simulink model "multi_opts"  (Simulink 4.00)
settings: Solver=ode45  SolverMode=SingleTasking  StartTime=0  StopTime=5  MaxStep=0.1  RelTol=1e-3  AbsTol=1e-3
libraries: simulink3 x3
(part 1 of 2)
settings Model: LastModifiedBy=mark  Refine=5  SaveTime=off  SaveOutput=off  LimitDataPoints=off  RTWTemplateMakefile=grt_unix.tmf

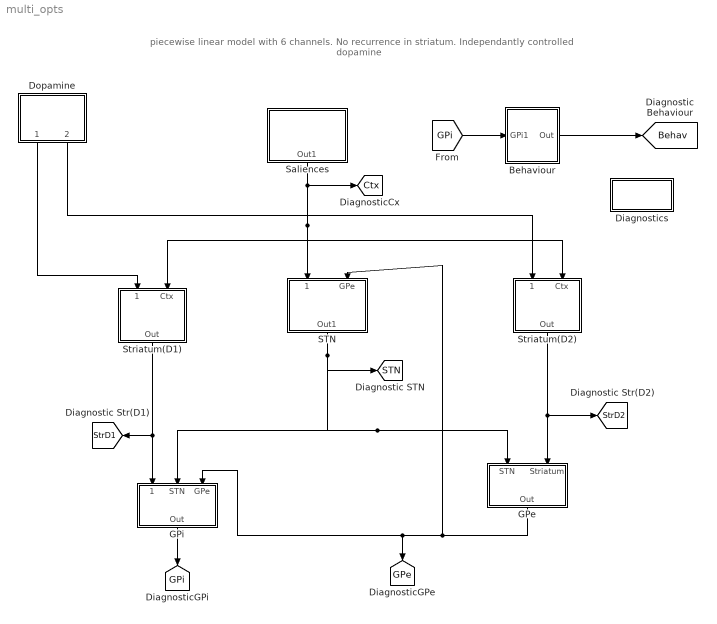
== system multi_opts ==
  note: piecewise linear model with 6 channels. No recurrence in
      | striatum. Independantly controlled dopamine
  Behaviour : Subsystem  mask(Behaviour expression){on_thresh=0.025, off_thresh=0.1}
      mask prompts: on_thresh "GPi level for behav. on"; off_thresh "GPi level for behav.  off"
      settings: RTWFcnNameOpts=Auto  RTWFileNameOpts=Auto
  Diagnostics : Subsystem
      settings: RTWFcnNameOpts=Auto  RTWFileNameOpts=Auto
  Dopamine : Subsystem  Orientation=down
      settings: RTWFcnNameOpts=Auto  RTWFileNameOpts=Auto
  GPe : Subsystem  Orientation=down  mask(GPe){W_str=-1, W_STN=0.8, A_rate=25, slope=1, thresh=-0.2}
      mask prompts: W_str "weight from Striatum"; W_STN "weight from STN (exc.)"; A_rate "membrane decay rate"; slope "output slope"; thresh "output thresh"
      mask help: 3 channel GPe
      settings: RTWFcnNameOpts=Auto  RTWFileNameOpts=Auto
  GPi : Subsystem  Orientation=down  mask(GPi){W_str=-1, W_STN=0.8, W_GPe=-0.4, A_rate=25, slope=1, thresh=-0.2}
      mask prompts: W_str "weight from Str"; W_STN "weight from STN"; W_GPe "weight from GPe"; A_rate "membrane decay rate"; slope "output slope"; thresh "output thresh"
      mask help: 3 channel GPe
      settings: RTWFcnNameOpts=Auto  RTWFileNameOpts=Auto
  STN : Subsystem  Orientation=down
      settings: RTWFcnNameOpts=Auto  RTWFileNameOpts=Auto
  Saliences : Subsystem  Orientation=down
      settings: RTWFcnNameOpts=Auto  RTWFileNameOpts=Auto
  Striatum(D1) : Subsystem  Orientation=down  mask(Striatum (D1)){W_ext=1, A_rate=25, slope=1, thresh=0.2}
      mask prompts: W_ext "External input weight"; A_rate "membrane decay rate"; slope "output slope"; thresh "output thresh"
      mask help: 3 channel striatum - non-recurrent
      settings: RTWFcnNameOpts=Auto  RTWFileNameOpts=Auto
  Striatum(D2) : Subsystem  Orientation=down  mask(Striatum (D1)){W_ext=1, A_rate=25, slope=1, thresh=0.2}
      mask prompts: W_ext "External input weight"; A_rate "membrane decay rate"; slope "output slope"; thresh "output thresh"
      mask help: 3 channel striatum - non-recurrent
      settings: RTWFcnNameOpts=Auto  RTWFileNameOpts=Auto
  tag scope: Behav=global, Ctx=global, GPe=global, GPi=global, STN=global, StrD1=global, StrD2=global
  wires:
  Saliences/1(Out1) -> [Ctx], Striatum(D2)/2(Ctx), Striatum(D1)/2(Ctx), STN/1(salineces)
  [GPi] -> Behaviour/1(GPi1)
  Behaviour/1(Out) -> [Behav]
  GPe/1(Out) -> STN/2(GPe), GPi/3(GPe), [GPe]
  Striatum(D2)/1(Out) -> GPe/2(Striatum), [StrD2]
  STN/1(Out1) -> [STN], GPe/1(STN), GPi/2(STN)
  GPi/1(Out) -> [GPi]
  Striatum(D1)/1(Out) -> GPi/1(Striatum), [StrD1]
  Dopamine/2(GPe(D2)) -> Striatum(D2)/1(Dopamine)
  Dopamine/1(GPi(D1)) -> Striatum(D1)/1(Dopamine)

== system multi_opts/Behaviour ==
  GPi1 : Inport  Port=1  LatchInput=off
  Constant : Constant  Value=1
  Relay : Relay  OnSwitchValue=1 - on_thresh  OffSwitchValue=1 - off_thresh  OnOutputValue=1  OffOutputValue=0
  Sum : Sum  Inputs=+-  SaturateOnIntegerOverflow=on
  Out : Outport  Port=1  InitialOutput=0
  wires:
  Constant/1 -> Sum/1
  Sum/1 -> Relay/1
  GPi1/1 -> Sum/2
  Relay/1 -> Out/1

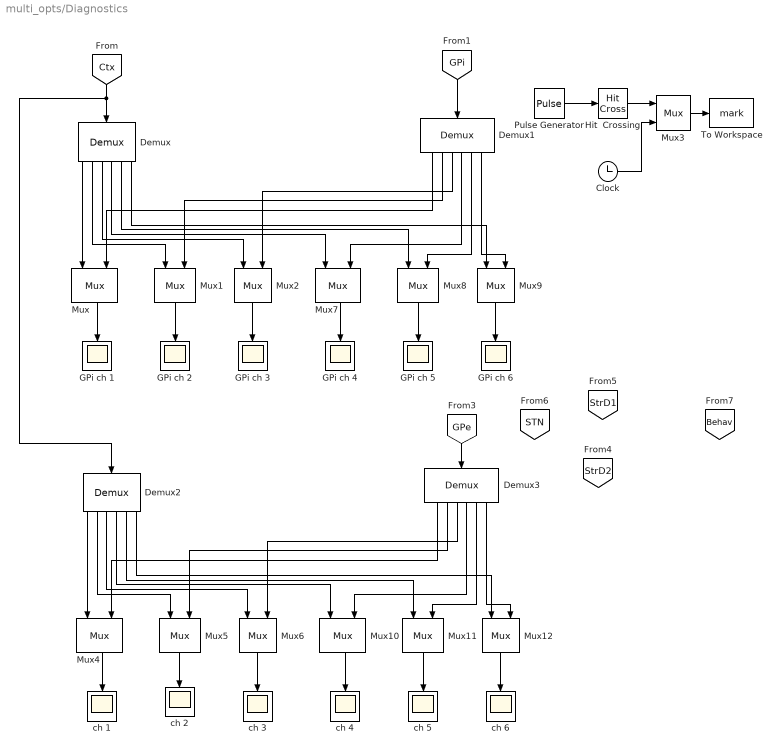
== system multi_opts/Diagnostics ==
  Clock : Clock
      settings: DisplayTime=off  Decimation=10
  Demux{,1..3} (4 alike) : Demux  Orientation=down  Outputs=6  BusSelectionMode=off
  GPi ch {1..6} (6 alike) : Scope
      GPi ch 1 settings: Orientation=down  TickLabels=on  TimeRange=auto  YMin=0  YMax=1  SaveName=GPic1_6  DataFormat=Array  LimitDataPoints=on  MaxDataPoints=7000
      GPi ch 2 settings: Orientation=down  TickLabels=on  TimeRange=auto  YMin=0  YMax=1  SaveName=GPic2_6  DataFormat=Array  LimitDataPoints=on  MaxDataPoints=7000
      GPi ch 3 settings: Orientation=down  TickLabels=on  TimeRange=auto  YMin=0  YMax=1  SaveName=GPic3_6  DataFormat=Array  LimitDataPoints=on  MaxDataPoints=5000
      GPi ch 4 settings: Orientation=down  TickLabels=on  TimeRange=auto  YMin=0  YMax=0.75  SaveToWorkspace=off  SaveName=GPic4_6  DataFormat=Array  LimitDataPoints=on  MaxDataPoints=5000
      GPi ch 5 settings: Orientation=down  TickLabels=on  TimeRange=auto  YMin=0  YMax=0.75  SaveToWorkspace=off  SaveName=GPi3full  DataFormat=Array  LimitDataPoints=on  MaxDataPoints=5000
      GPi ch 6 settings: Orientation=down  TickLabels=on  TimeRange=auto  YMin=0  YMax=0.75  SaveToWorkspace=off  SaveName=GPi6full6  DataFormat=Array  LimitDataPoints=on  MaxDataPoints=5000
  Hit  Crossing : HitCross  HitCrossingOffset=0.5  HitCrossingDirection=falling  ShowOutputPort=on
  Mux{,1..2,4..12} (12 alike) : Mux  Orientation=down  Inputs=2
      settings: DisplayOption=none
  Mux3 : Mux  Inputs=2
      settings: DisplayOption=none
  Pulse Generator : DiscretePulseGenerator  PulseType=Time-based  Amplitude=1  Period=0.5  PulseWidth=50  PhaseDelay=0.0  SampleTime=1
  To Workspace : ToWorkspace  VariableName=mark  SampleTime=-1  SaveFormat=Array
  ch {1..6} (6 alike) : Scope
      ch 1 settings: Orientation=down  TickLabels=on  TimeRange=auto  YMin=0  YMax=1  SaveName=gpe1  DataFormat=Array  LimitDataPoints=on  MaxDataPoints=5000
      ch 2 settings: Orientation=down  TickLabels=on  TimeRange=auto  YMin=0  YMax=0.75  SaveName=gpe2  DataFormat=Array  LimitDataPoints=on  MaxDataPoints=5000
      ch 3 settings: Orientation=down  TickLabels=on  TimeRange=auto  YMin=0  YMax=0.75  SaveToWorkspace=off  SaveName=ch3  DataFormat=Array  LimitDataPoints=on  MaxDataPoints=5000
      ch 4 settings: Orientation=down  TickLabels=on  TimeRange=auto  YMin=0  YMax=0.75  SaveToWorkspace=off  SaveName=ch4  DataFormat=Array  LimitDataPoints=on  MaxDataPoints=5000
      ch 5 settings: Orientation=down  TickLabels=on  TimeRange=auto  YMin=0  YMax=0.75  SaveToWorkspace=off  SaveName=ch5  DataFormat=Array  LimitDataPoints=on  MaxDataPoints=5000
      ch 6 settings: Orientation=down  TickLabels=on  TimeRange=auto  YMin=0  YMax=0.75  SaveToWorkspace=off  SaveName=ch6  DataFormat=Array  LimitDataPoints=on  MaxDataPoints=5000
  wires:
  [GPe] -> Demux3/1
  Mux/1 -> GPi ch 1/1
  Demux/1 -> Mux/1
  Demux/2 -> Mux1/1
  Mux1/1 -> GPi ch 2/1
  Mux2/1 -> GPi ch 3/1
  Demux/3 -> Mux2/1
  Demux/4 -> Mux7/1
  Demux/5 -> Mux8/1
  Demux/6 -> Mux9/1
  Demux1/3 -> Mux2/2
  [GPi] -> Demux1/1
  Demux1/1 -> Mux/2
  Demux1/2 -> Mux1/2
  Demux1/4 -> Mux7/2
  Demux1/5 -> Mux8/2
  Demux1/6 -> Mux9/2
  Mux7/1 -> GPi ch 4/1
  Mux8/1 -> GPi ch 5/1
  Mux9/1 -> GPi ch 6/1
  [Ctx] -> Demux/1, Demux2/1
  Mux4/1 -> ch 1/1
  Demux2/1 -> Mux4/1
  Demux2/2 -> Mux5/1
  Mux5/1 -> ch 2/1
  Mux6/1 -> ch 3/1
  Demux2/3 -> Mux6/1
  Demux2/4 -> Mux10/1
  Demux2/5 -> Mux11/1
  Demux2/6 -> Mux12/1
  Demux3/3 -> Mux6/2
  Demux3/1 -> Mux4/2
  Demux3/2 -> Mux5/2
  Demux3/4 -> Mux10/2
  Demux3/5 -> Mux11/2
  Demux3/6 -> Mux12/2
  Mux10/1 -> ch 4/1
  Mux11/1 -> ch 5/1
  Mux12/1 -> ch 6/1
  Pulse Generator/1 -> Hit  Crossing/1
  Hit  Crossing/1 -> Mux3/1
  Clock/1 -> Mux3/2
  Mux3/1 -> To Workspace/1

== system multi_opts/Dopamine ==
  D1 base level : Constant  Value=0.2
  D2 base level : Constant  Orientation=left  Value=0.2
  Mux : Mux  Orientation=down  Inputs=6
      settings: DisplayOption=none
  Mux1 : Mux  Orientation=down  Inputs=6
      settings: DisplayOption=none
  GPi(D1) : Outport  Orientation=down  Port=1  InitialOutput=0
  GPe(D2) : Outport  Orientation=down  Port=2  InitialOutput=0
  wires:
  Mux1/1 -> GPe(D2)/1
  D2 base level/1 -> Mux1/6, Mux1/5, Mux1/4, Mux1/3, Mux1/2, Mux1/1
  Mux/1 -> GPi(D1)/1
  D1 base level/1 -> Mux/6, Mux/5, Mux/4, Mux/3, Mux/2, Mux/1

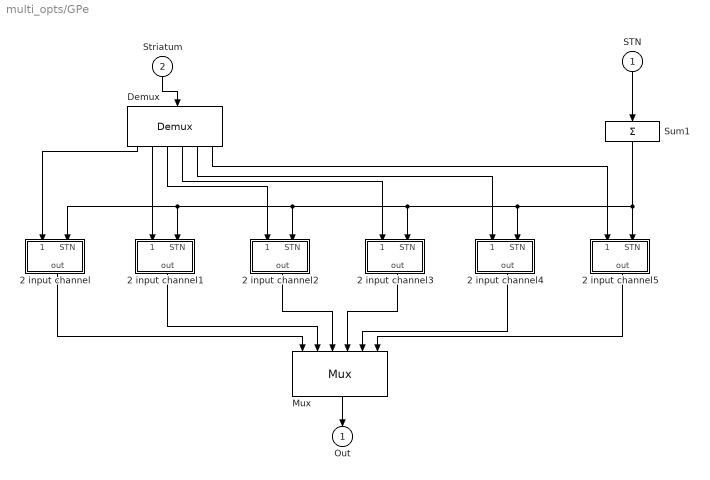
== system multi_opts/GPe ==
  STN : Inport  Orientation=down  Port=1  LatchInput=off
  Striatum : Inport  Orientation=down  Port=2  LatchInput=off
  2 input channel : Subsystem  Orientation=down
      settings: RTWFcnNameOpts=Auto  RTWFileNameOpts=Auto
  2 input channel1 : Subsystem  Orientation=down
      settings: RTWFcnNameOpts=Auto  RTWFileNameOpts=Auto
  2 input channel2 : Subsystem  Orientation=down
      settings: RTWFcnNameOpts=Auto  RTWFileNameOpts=Auto
  2 input channel3 : Subsystem  Orientation=down
      settings: RTWFcnNameOpts=Auto  RTWFileNameOpts=Auto
  2 input channel4 : Subsystem  Orientation=down
      settings: RTWFcnNameOpts=Auto  RTWFileNameOpts=Auto
  2 input channel5 : Subsystem  Orientation=down
      settings: RTWFcnNameOpts=Auto  RTWFileNameOpts=Auto
  Demux : Demux  Orientation=down  Outputs=6  BusSelectionMode=off
  Mux : Mux  Orientation=down  Inputs=6
      settings: DisplayOption=none
  Sum1 : Sum  Orientation=down  Inputs=+  SaturateOnIntegerOverflow=on
  Out : Outport  Orientation=down  Port=1  InitialOutput=0
  wires:
  Sum1/1 -> 2 input channel5/2(STN), 2 input channel/2(STN), 2 input channel1/2(STN), 2 input channel2/2(STN), 2 input channel3/2(STN), 2 input channel4/2(STN)
  Demux/1 -> 2 input channel/1(Striatum)
  STN/1 -> Sum1/1
  2 input channel/1(out) -> Mux/1
  2 input channel1/1(out) -> Mux/2
  2 input channel2/1(out) -> Mux/3
  Mux/1 -> Out/1
  Striatum/1 -> Demux/1
  Demux/2 -> 2 input channel1/1(Striatum)
  Demux/3 -> 2 input channel2/1(Striatum)
  Demux/4 -> 2 input channel3/1(Striatum)
  Demux/5 -> 2 input channel4/1(Striatum)
  Demux/6 -> 2 input channel5/1(Striatum)
  2 input channel3/1(out) -> Mux/4
  2 input channel4/1(out) -> Mux/5
  2 input channel5/1(out) -> Mux/6

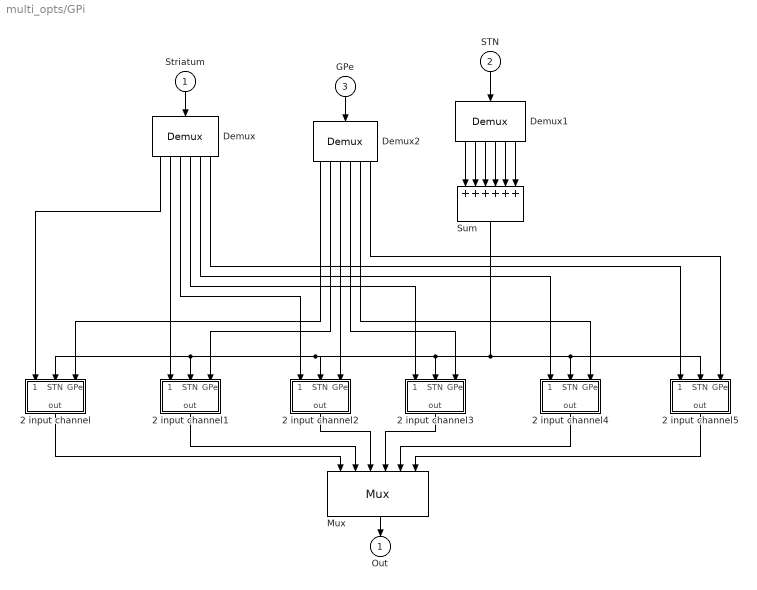
== system multi_opts/GPi ==
  Striatum : Inport  Orientation=down  Port=1  LatchInput=off
  STN : Inport  Orientation=down  Port=2  LatchInput=off
  GPe : Inport  Orientation=down  Port=3  LatchInput=off
  2 input channel : Subsystem  Orientation=down
      settings: RTWFcnNameOpts=Auto  RTWFileNameOpts=Auto
  2 input channel1 : Subsystem  Orientation=down
      settings: RTWFcnNameOpts=Auto  RTWFileNameOpts=Auto
  2 input channel2 : Subsystem  Orientation=down
      settings: RTWFcnNameOpts=Auto  RTWFileNameOpts=Auto
  2 input channel3 : Subsystem  Orientation=down
      settings: RTWFcnNameOpts=Auto  RTWFileNameOpts=Auto
  2 input channel4 : Subsystem  Orientation=down
      settings: RTWFcnNameOpts=Auto  RTWFileNameOpts=Auto
  2 input channel5 : Subsystem  Orientation=down
      settings: RTWFcnNameOpts=Auto  RTWFileNameOpts=Auto
  Demux : Demux  Orientation=down  Outputs=6  BusSelectionMode=off
  Demux1 : Demux  Orientation=down  Outputs=6  BusSelectionMode=off
  Demux2 : Demux  Orientation=down  Outputs=6  BusSelectionMode=off
  Mux : Mux  Orientation=down  Inputs=6
      settings: DisplayOption=none
  Sum : Sum  Orientation=down  Inputs=++++++  SaturateOnIntegerOverflow=on
  Out : Outport  Orientation=down  Port=1  InitialOutput=0
  wires:
  Mux/1 -> Out/1
  2 input channel2/1(out) -> Mux/3
  2 input channel1/1(out) -> Mux/2
  2 input channel/1(out) -> Mux/1
  GPe/1 -> Demux2/1
  Demux2/1 -> 2 input channel/3(GPe)
  Demux2/2 -> 2 input channel1/3(GPe)
  Demux2/3 -> 2 input channel2/3(GPe)
  Demux/2 -> 2 input channel1/1(Striatum)
  Demux/1 -> 2 input channel/1(Striatum)
  Striatum/1 -> Demux/1
  Demux/3 -> 2 input channel2/1(Striatum)
  Demux/4 -> 2 input channel3/1(Striatum)
  Demux/5 -> 2 input channel4/1(Striatum)
  Demux/6 -> 2 input channel5/1(Striatum)
  Demux2/4 -> 2 input channel3/3(GPe)
  Demux2/5 -> 2 input channel4/3(GPe)
  Demux1/1 -> Sum/1
  Demux1/2 -> Sum/2
  Demux1/3 -> Sum/3
  Demux1/4 -> Sum/4
  Demux1/5 -> Sum/5
  Demux1/6 -> Sum/6
  STN/1 -> Demux1/1
  Sum/1 -> 2 input channel/2(STN), 2 input channel1/2(STN), 2 input channel2/2(STN), 2 input channel3/2(STN), 2 input channel4/2(STN), 2 input channel5/2(STN)
  Demux2/6 -> 2 input channel5/3(GPe)
  2 input channel3/1(out) -> Mux/4
  2 input channel4/1(out) -> Mux/5
  2 input channel5/1(out) -> Mux/6

== system multi_opts/STN ==
  salineces : Inport  Orientation=down  Port=1  LatchInput=off
  GPe : Inport  Orientation=down  Port=2  LatchInput=off
  Do discrete STN : Constant  Orientation=down  Value=1
  STN discrete model : Subsystem  Orientation=down  mask(STN){W_ctx=1, W_GPe=-1, A_rate=25, slope=1, thresh=-0.25}
      mask prompts: W_ctx "weight from Cortex"; W_GPe "weight from GPe(inhib.)"; A_rate "membrane decay rate"; slope "output slope"; thresh "output thresh"
      mask help: 3 channel GPe
      settings: RTWFcnNameOpts=Auto  RTWFileNameOpts=Auto
  STN homogeneous model : Subsystem  Orientation=down  mask(STN){epsilon_p=0.25, W_ctx=1, W_GPe=-1, A_rate=25, slope=1, thresh=0}
      mask prompts: epsilon_p "Ctx tonic rate (per channel)"; W_ctx "weight from Ctx"; W_GPe "weight from GPe(inhib.)"; A_rate "membrane decay rate"; slope "output slope"; thresh "output thresh"
      mask help: 3 channel GPe
      settings: RTWFcnNameOpts=Auto  RTWFileNameOpts=Auto
  Switch1 : Switch  Orientation=down  Threshold=0.5
  Out1 : Outport  Orientation=down  Port=1  InitialOutput=0
  wires:
  STN homogeneous model/1(Out) -> Switch1/3
  GPe/1 -> STN discrete model/2(GPe), STN homogeneous model/2(GPe)
  salineces/1 -> STN homogeneous model/1(Cortex), STN discrete model/1(Cortex)
  Switch1/1 -> Out1/1
  Do discrete STN/1 -> Switch1/2
  STN discrete model/1(Out) -> Switch1/1

== system multi_opts/Saliences ==
  Do left : Constant  Orientation=down  Value=0
  Salience (simple) : Subsystem  Orientation=down
      settings: RTWFcnNameOpts=Auto  RTWFileNameOpts=Auto
  Switch : Switch  Orientation=down  Threshold=0.5
  step pairs : Subsystem  Orientation=down
      settings: RTWFcnNameOpts=Auto  RTWFileNameOpts=Auto
  Out1 : Outport  Orientation=down  Port=1  InitialOutput=0
  wires:
  Switch/1 -> Out1/1
  Salience (simple)/1(out) -> Switch/3
  step pairs/1(out) -> Switch/1
  Do left/1 -> Switch/2

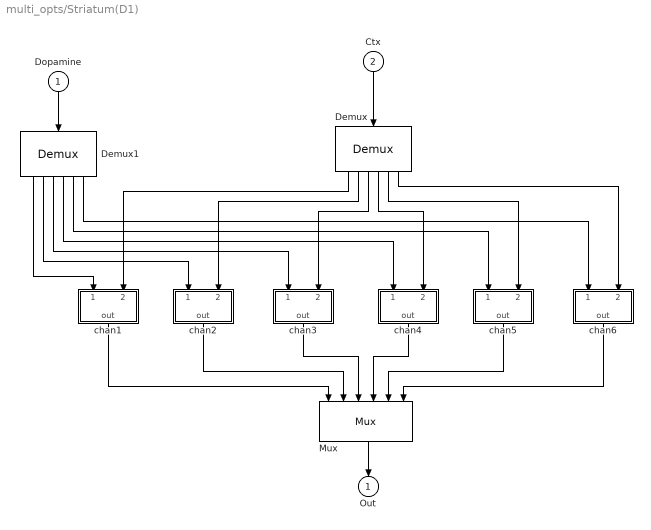
== system multi_opts/Striatum(D1) ==
  Dopamine : Inport  Orientation=down  Port=1  LatchInput=off
  Ctx : Inport  Orientation=down  Port=2  LatchInput=off
  Demux : Demux  Orientation=down  Outputs=6  BusSelectionMode=off
  Demux1 : Demux  Orientation=down  Outputs=6  BusSelectionMode=off
  Mux : Mux  Orientation=down  Inputs=6
      settings: DisplayOption=none
  chan1 : Subsystem  Orientation=down
      settings: RTWFcnNameOpts=Auto  RTWFileNameOpts=Auto
  chan2 : Subsystem  Orientation=down
      settings: RTWFcnNameOpts=Auto  RTWFileNameOpts=Auto
  chan3 : Subsystem  Orientation=down
      settings: RTWFcnNameOpts=Auto  RTWFileNameOpts=Auto
  chan4 : Subsystem  Orientation=down
      settings: RTWFcnNameOpts=Auto  RTWFileNameOpts=Auto
  chan5 : Subsystem  Orientation=down
      settings: RTWFcnNameOpts=Auto  RTWFileNameOpts=Auto
  chan6 : Subsystem  Orientation=down
      settings: RTWFcnNameOpts=Auto  RTWFileNameOpts=Auto
  Out : Outport  Orientation=down  Port=1  InitialOutput=0
  wires:
  Ctx/1 -> Demux/1
  Mux/1 -> Out/1
  chan1/1(out) -> Mux/1
  chan3/1(out) -> Mux/3
  chan2/1(out) -> Mux/2
  Demux/1 -> chan1/2(external)
  Demux/2 -> chan2/2(external)
  Demux/3 -> chan3/2(external)
  Demux/4 -> chan4/2(external)
  Demux/5 -> chan5/2(external)
  Demux/6 -> chan6/2(external)
  chan4/1(out) -> Mux/4
  chan5/1(out) -> Mux/5
  chan6/1(out) -> Mux/6
  Dopamine/1 -> Demux1/1
  Demux1/6 -> chan6/1(dopamine)
  Demux1/5 -> chan5/1(dopamine)
  Demux1/4 -> chan4/1(dopamine)
  Demux1/3 -> chan3/1(dopamine)
  Demux1/2 -> chan2/1(dopamine)
  Demux1/1 -> chan1/1(dopamine)

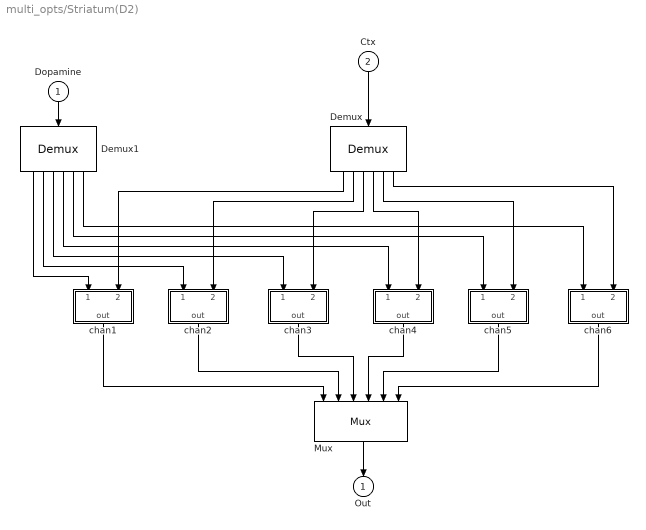
== system multi_opts/Striatum(D2) ==
  Dopamine : Inport  Orientation=down  Port=1  LatchInput=off
  Ctx : Inport  Orientation=down  Port=2  LatchInput=off
  Demux : Demux  Orientation=down  Outputs=6  BusSelectionMode=off
  Demux1 : Demux  Orientation=down  Outputs=6  BusSelectionMode=off
  Mux : Mux  Orientation=down  Inputs=6
      settings: DisplayOption=none
  chan1 : Subsystem  Orientation=down
      settings: RTWFcnNameOpts=Auto  RTWFileNameOpts=Auto
  chan2 : Subsystem  Orientation=down
      settings: RTWFcnNameOpts=Auto  RTWFileNameOpts=Auto
  chan3 : Subsystem  Orientation=down
      settings: RTWFcnNameOpts=Auto  RTWFileNameOpts=Auto
  chan4 : Subsystem  Orientation=down
      settings: RTWFcnNameOpts=Auto  RTWFileNameOpts=Auto
  chan5 : Subsystem  Orientation=down
      settings: RTWFcnNameOpts=Auto  RTWFileNameOpts=Auto
  chan6 : Subsystem  Orientation=down
      settings: RTWFcnNameOpts=Auto  RTWFileNameOpts=Auto
  Out : Outport  Orientation=down  Port=1  InitialOutput=0
  wires:
  chan6/1(out) -> Mux/6
  chan5/1(out) -> Mux/5
  chan4/1(out) -> Mux/4
  Demux/6 -> chan6/2(external)
  Demux/5 -> chan5/2(external)
  Demux/4 -> chan4/2(external)
  Demux/3 -> chan3/2(external)
  Demux/2 -> chan2/2(external)
  Demux/1 -> chan1/2(external)
  chan2/1(out) -> Mux/2
  chan3/1(out) -> Mux/3
  chan1/1(out) -> Mux/1
  Mux/1 -> Out/1
  Ctx/1 -> Demux/1
  Dopamine/1 -> Demux1/1
  Demux1/6 -> chan6/1(dopamine)
  Demux1/5 -> chan5/1(dopamine)
  Demux1/4 -> chan4/1(dopamine)
  Demux1/3 -> chan3/1(dopamine)
  Demux1/2 -> chan2/1(dopamine)
  Demux1/1 -> chan1/1(dopamine)

== system multi_opts/GPe/2 input channel ==
  Striatum : Inport  Orientation=down  Port=1  LatchInput=off
  STN : Inport  Orientation=down  Port=2  LatchInput=off
  input summation : Subsystem  Orientation=down
      settings: RTWFcnNameOpts=Auto  RTWFileNameOpts=Auto
  leaky integration : Subsystem  Orientation=down
      settings: RTWFcnNameOpts=Auto  RTWFileNameOpts=Auto
  piecewise lin. : S-Function  Orientation=down  FunctionName=Mpieclin  Parameters=slope,thresh  PortCounts=[]  SFunctionModules=''
  out : Outport  Orientation=down  Port=1  InitialOutput=0
  wires:
  leaky integration/1(Outport) -> piecewise lin./1
  input summation/1(out_1) -> leaky integration/1(Inport)
  Striatum/1 -> input summation/1(x1)
  STN/1 -> input summation/2(x2)
  piecewise lin./1 -> out/1

== system multi_opts/GPe/2 input channel1 ==
  Striatum : Inport  Orientation=down  Port=1  LatchInput=off
  STN : Inport  Orientation=down  Port=2  LatchInput=off
  input summation : Subsystem  Orientation=down
      settings: RTWFcnNameOpts=Auto  RTWFileNameOpts=Auto
  leaky integration : Subsystem  Orientation=down
      settings: RTWFcnNameOpts=Auto  RTWFileNameOpts=Auto
  piecewise lin. : S-Function  Orientation=down  FunctionName=Mpieclin  Parameters=slope,thresh  PortCounts=[]  SFunctionModules=''
  out : Outport  Orientation=down  Port=1  InitialOutput=0
  wires:
  piecewise lin./1 -> out/1
  STN/1 -> input summation/2(x2)
  Striatum/1 -> input summation/1(x1)
  leaky integration/1(Outport) -> piecewise lin./1
  input summation/1(out_1) -> leaky integration/1(Inport)

== system multi_opts/GPe/2 input channel2 ==
  Striatum : Inport  Orientation=down  Port=1  LatchInput=off
  STN : Inport  Orientation=down  Port=2  LatchInput=off
  input summation : Subsystem  Orientation=down
      settings: RTWFcnNameOpts=Auto  RTWFileNameOpts=Auto
  leaky integration : Subsystem  Orientation=down
      settings: RTWFcnNameOpts=Auto  RTWFileNameOpts=Auto
  piecewise lin. : S-Function  Orientation=down  FunctionName=Mpieclin  Parameters=slope,thresh  PortCounts=[]  SFunctionModules=''
  out : Outport  Orientation=down  Port=1  InitialOutput=0
  wires:
  input summation/1(out_1) -> leaky integration/1(Inport)
  leaky integration/1(Outport) -> piecewise lin./1
  Striatum/1 -> input summation/1(x1)
  STN/1 -> input summation/2(x2)
  piecewise lin./1 -> out/1

== system multi_opts/GPe/2 input channel3 ==
  Striatum : Inport  Orientation=down  Port=1  LatchInput=off
  STN : Inport  Orientation=down  Port=2  LatchInput=off
  input summation : Subsystem  Orientation=down
      settings: RTWFcnNameOpts=Auto  RTWFileNameOpts=Auto
  leaky integration : Subsystem  Orientation=down
      settings: RTWFcnNameOpts=Auto  RTWFileNameOpts=Auto
  piecewise lin. : S-Function  Orientation=down  FunctionName=Mpieclin  Parameters=slope,thresh  PortCounts=[]  SFunctionModules=''
  out : Outport  Orientation=down  Port=1  InitialOutput=0
  wires:
  piecewise lin./1 -> out/1
  STN/1 -> input summation/2(x2)
  Striatum/1 -> input summation/1(x1)
  leaky integration/1(Outport) -> piecewise lin./1
  input summation/1(out_1) -> leaky integration/1(Inport)

== system multi_opts/GPe/2 input channel4 ==
  Striatum : Inport  Orientation=down  Port=1  LatchInput=off
  STN : Inport  Orientation=down  Port=2  LatchInput=off
  input summation : Subsystem  Orientation=down
      settings: RTWFcnNameOpts=Auto  RTWFileNameOpts=Auto
  leaky integration : Subsystem  Orientation=down
      settings: RTWFcnNameOpts=Auto  RTWFileNameOpts=Auto
  piecewise lin. : S-Function  Orientation=down  FunctionName=Mpieclin  Parameters=slope,thresh  PortCounts=[]  SFunctionModules=''
  out : Outport  Orientation=down  Port=1  InitialOutput=0
  wires:
  input summation/1(out_1) -> leaky integration/1(Inport)
  leaky integration/1(Outport) -> piecewise lin./1
  Striatum/1 -> input summation/1(x1)
  STN/1 -> input summation/2(x2)
  piecewise lin./1 -> out/1

== system multi_opts/GPe/2 input channel5 ==
  Striatum : Inport  Orientation=down  Port=1  LatchInput=off
  STN : Inport  Orientation=down  Port=2  LatchInput=off
  input summation : Subsystem  Orientation=down
      settings: RTWFcnNameOpts=Auto  RTWFileNameOpts=Auto
  leaky integration : Subsystem  Orientation=down
      settings: RTWFcnNameOpts=Auto  RTWFileNameOpts=Auto
  piecewise lin. : S-Function  Orientation=down  FunctionName=Mpieclin  Parameters=slope,thresh  PortCounts=[]  SFunctionModules=''
  out : Outport  Orientation=down  Port=1  InitialOutput=0
  wires:
  piecewise lin./1 -> out/1
  STN/1 -> input summation/2(x2)
  Striatum/1 -> input summation/1(x1)
  leaky integration/1(Outport) -> piecewise lin./1
  input summation/1(out_1) -> leaky integration/1(Inport)

== system multi_opts/GPi/2 input channel ==
  Striatum : Inport  Orientation=down  Port=1  LatchInput=off
  STN : Inport  Orientation=down  Port=2  LatchInput=off
  GPe : Inport  Orientation=down  Port=3  LatchInput=off
  input summation : Subsystem  Orientation=down
      settings: RTWFcnNameOpts=Auto  RTWFileNameOpts=Auto
  leaky integration : Subsystem  Orientation=down
      settings: RTWFcnNameOpts=Auto  RTWFileNameOpts=Auto
  piecewise lin. : S-Function  Orientation=down  FunctionName=Mpieclin  Parameters=slope,thresh  PortCounts=[]  SFunctionModules=''
  out : Outport  Orientation=down  Port=1  InitialOutput=0
  wires:
  piecewise lin./1 -> out/1
  STN/1 -> input summation/2(x2)
  Striatum/1 -> input summation/1(x1)
  leaky integration/1(Outport) -> piecewise lin./1
  input summation/1(out_1) -> leaky integration/1(Inport)
  GPe/1 -> input summation/3(x3)

== system multi_opts/GPi/2 input channel1 ==
  Striatum : Inport  Orientation=down  Port=1  LatchInput=off
  STN : Inport  Orientation=down  Port=2  LatchInput=off
  GPe : Inport  Orientation=down  Port=3  LatchInput=off
  input summation : Subsystem  Orientation=down
      settings: RTWFcnNameOpts=Auto  RTWFileNameOpts=Auto
  leaky integration : Subsystem  Orientation=down
      settings: RTWFcnNameOpts=Auto  RTWFileNameOpts=Auto
  piecewise lin. : S-Function  Orientation=down  FunctionName=Mpieclin  Parameters=slope,thresh  PortCounts=[]  SFunctionModules=''
  out : Outport  Orientation=down  Port=1  InitialOutput=0
  wires:
  GPe/1 -> input summation/3(x3)
  input summation/1(out_1) -> leaky integration/1(Inport)
  leaky integration/1(Outport) -> piecewise lin./1
  Striatum/1 -> input summation/1(x1)
  STN/1 -> input summation/2(x2)
  piecewise lin./1 -> out/1

== system multi_opts/GPi/2 input channel2 ==
  Striatum : Inport  Orientation=down  Port=1  LatchInput=off
  STN : Inport  Orientation=down  Port=2  LatchInput=off
  GPe : Inport  Orientation=down  Port=3  LatchInput=off
  input summation : Subsystem  Orientation=down
      settings: RTWFcnNameOpts=Auto  RTWFileNameOpts=Auto
  leaky integration : Subsystem  Orientation=down
      settings: RTWFcnNameOpts=Auto  RTWFileNameOpts=Auto
  piecewise lin. : S-Function  Orientation=down  FunctionName=Mpieclin  Parameters=slope,thresh  PortCounts=[]  SFunctionModules=''
  out : Outport  Orientation=down  Port=1  InitialOutput=0
  wires:
  piecewise lin./1 -> out/1
  STN/1 -> input summation/2(x2)
  Striatum/1 -> input summation/1(x1)
  leaky integration/1(Outport) -> piecewise lin./1
  input summation/1(out_1) -> leaky integration/1(Inport)
  GPe/1 -> input summation/3(x3)

== system multi_opts/GPi/2 input channel3 ==
  Striatum : Inport  Orientation=down  Port=1  LatchInput=off
  STN : Inport  Orientation=down  Port=2  LatchInput=off
  GPe : Inport  Orientation=down  Port=3  LatchInput=off
  input summation : Subsystem  Orientation=down
      settings: RTWFcnNameOpts=Auto  RTWFileNameOpts=Auto
  leaky integration : Subsystem  Orientation=down
      settings: RTWFcnNameOpts=Auto  RTWFileNameOpts=Auto
  piecewise lin. : S-Function  Orientation=down  FunctionName=Mpieclin  Parameters=slope,thresh  PortCounts=[]  SFunctionModules=''
  out : Outport  Orientation=down  Port=1  InitialOutput=0
  wires:
  GPe/1 -> input summation/3(x3)
  input summation/1(out_1) -> leaky integration/1(Inport)
  leaky integration/1(Outport) -> piecewise lin./1
  Striatum/1 -> input summation/1(x1)
  STN/1 -> input summation/2(x2)
  piecewise lin./1 -> out/1

== system multi_opts/GPi/2 input channel4 ==
  Striatum : Inport  Orientation=down  Port=1  LatchInput=off
  STN : Inport  Orientation=down  Port=2  LatchInput=off
  GPe : Inport  Orientation=down  Port=3  LatchInput=off
  input summation : Subsystem  Orientation=down
      settings: RTWFcnNameOpts=Auto  RTWFileNameOpts=Auto
  leaky integration : Subsystem  Orientation=down
      settings: RTWFcnNameOpts=Auto  RTWFileNameOpts=Auto
  piecewise lin. : S-Function  Orientation=down  FunctionName=Mpieclin  Parameters=slope,thresh  PortCounts=[]  SFunctionModules=''
  out : Outport  Orientation=down  Port=1  InitialOutput=0
  wires:
  piecewise lin./1 -> out/1
  STN/1 -> input summation/2(x2)
  Striatum/1 -> input summation/1(x1)
  leaky integration/1(Outport) -> piecewise lin./1
  input summation/1(out_1) -> leaky integration/1(Inport)
  GPe/1 -> input summation/3(x3)

== system multi_opts/GPi/2 input channel5 ==
  Striatum : Inport  Orientation=down  Port=1  LatchInput=off
  STN : Inport  Orientation=down  Port=2  LatchInput=off
  GPe : Inport  Orientation=down  Port=3  LatchInput=off
  input summation : Subsystem  Orientation=down
      settings: RTWFcnNameOpts=Auto  RTWFileNameOpts=Auto
  leaky integration : Subsystem  Orientation=down
      settings: RTWFcnNameOpts=Auto  RTWFileNameOpts=Auto
  piecewise lin. : S-Function  Orientation=down  FunctionName=Mpieclin  Parameters=slope,thresh  PortCounts=[]  SFunctionModules=''
  out : Outport  Orientation=down  Port=1  InitialOutput=0
  wires:
  GPe/1 -> input summation/3(x3)
  input summation/1(out_1) -> leaky integration/1(Inport)
  leaky integration/1(Outport) -> piecewise lin./1
  Striatum/1 -> input summation/1(x1)
  STN/1 -> input summation/2(x2)
  piecewise lin./1 -> out/1

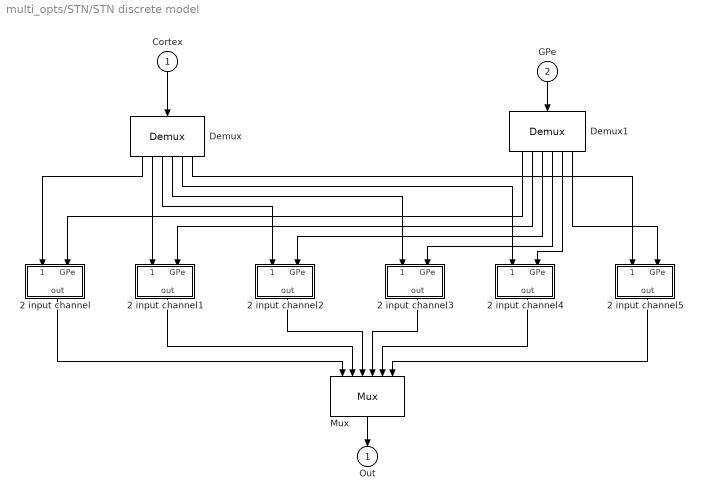
== system multi_opts/STN/STN discrete model ==
  Cortex : Inport  Orientation=down  Port=1  LatchInput=off
  GPe : Inport  Orientation=down  Port=2  LatchInput=off
  2 input channel : Subsystem  Orientation=down
      settings: RTWFcnNameOpts=Auto  RTWFileNameOpts=Auto
  2 input channel1 : Subsystem  Orientation=down
      settings: RTWFcnNameOpts=Auto  RTWFileNameOpts=Auto
  2 input channel2 : Subsystem  Orientation=down
      settings: RTWFcnNameOpts=Auto  RTWFileNameOpts=Auto
  2 input channel3 : Subsystem  Orientation=down
      settings: RTWFcnNameOpts=Auto  RTWFileNameOpts=Auto
  2 input channel4 : Subsystem  Orientation=down
      settings: RTWFcnNameOpts=Auto  RTWFileNameOpts=Auto
  2 input channel5 : Subsystem  Orientation=down
      settings: RTWFcnNameOpts=Auto  RTWFileNameOpts=Auto
  Demux : Demux  Orientation=down  Outputs=6  BusSelectionMode=off
  Demux1 : Demux  Orientation=down  Outputs=6  BusSelectionMode=off
  Mux : Mux  Orientation=down  Inputs=6
      settings: DisplayOption=none
  Out : Outport  Orientation=down  Port=1  InitialOutput=0
  wires:
  Demux/3 -> 2 input channel2/1(Cortex)
  Demux/2 -> 2 input channel1/1(Cortex)
  Demux/1 -> 2 input channel/1(Cortex)
  Cortex/1 -> Demux/1
  Mux/1 -> Out/1
  2 input channel2/1(out) -> Mux/3
  2 input channel1/1(out) -> Mux/2
  2 input channel/1(out) -> Mux/1
  2 input channel3/1(out) -> Mux/4
  2 input channel4/1(out) -> Mux/5
  2 input channel5/1(out) -> Mux/6
  Demux/4 -> 2 input channel3/1(Cortex)
  Demux/5 -> 2 input channel4/1(Cortex)
  Demux/6 -> 2 input channel5/1(Cortex)
  GPe/1 -> Demux1/1
  Demux1/1 -> 2 input channel/2(GPe)
  Demux1/2 -> 2 input channel1/2(GPe)
  Demux1/3 -> 2 input channel2/2(GPe)
  Demux1/4 -> 2 input channel3/2(GPe)
  Demux1/5 -> 2 input channel4/2(GPe)
  Demux1/6 -> 2 input channel5/2(GPe)

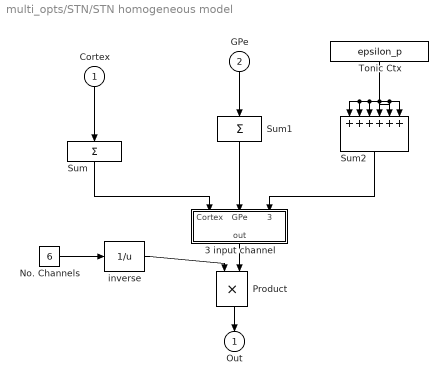
== system multi_opts/STN/STN homogeneous model ==
  Cortex : Inport  Orientation=down  Port=1  LatchInput=off
  GPe : Inport  Orientation=down  Port=2  LatchInput=off
  3 input channel : Subsystem  Orientation=down
      settings: RTWFcnNameOpts=Auto  RTWFileNameOpts=Auto
  No. Channels : Constant  Value=6
  Product : Product  Orientation=down  Inputs=2  Multiplication=Element-wise(.*)  SaturateOnIntegerOverflow=on
  Sum : Sum  Orientation=down  Inputs=+  SaturateOnIntegerOverflow=on
  Sum1 : Sum  Orientation=down  Inputs=+  SaturateOnIntegerOverflow=on
  Sum2 : Sum  Orientation=down  Inputs=++++++  SaturateOnIntegerOverflow=on
  Tonic Ctx : Constant  Orientation=down  Value=epsilon_p
  inverse : Fcn  Expr=1/u
  Out : Outport  Orientation=down  Port=1  InitialOutput=0
  wires:
  Sum1/1 -> 3 input channel/2(GPe)
  Product/1 -> Out/1
  No. Channels/1 -> inverse/1
  inverse/1 -> Product/1
  3 input channel/1(out) -> Product/2
  Sum/1 -> 3 input channel/1(Cortex)
  Sum2/1 -> 3 input channel/3(Tonic Ctx)
  GPe/1 -> Sum1/1
  Cortex/1 -> Sum/1
  Tonic Ctx/1 -> Sum2/6, Sum2/5, Sum2/4, Sum2/3, Sum2/2, Sum2/1

== system multi_opts/Saliences/Salience (simple) ==
  6 Saliences : DiscretePulseGenerator  Orientation=down  PulseType=Time-based  Amplitude=[0.4 0.6 0 0 0 0]  Period=10  PulseWidth=[90 90 10 10 10 10]  PhaseDelay=[1 2 4 10 10 10]  SampleTime=1
  Aux steps : DiscretePulseGenerator  Orientation=down  PulseType=Time-based  Amplitude=[0.2 0.0 0 0 0 0]  Period=10  PulseWidth=[10 10 10 10 10 10]  PhaseDelay=[3 10 10 10 10 10]  SampleTime=1
  Constant : Constant  Value=[0 0 0 0 0]
  Mux : Mux  Inputs=2
      settings: DisplayOption=none
  Repeating Sequence : simulink3/Sources/Repeating Sequence  rep_seq_t=[0 1 1.1 1.2 1.3 1.4 1.5 1.6 2 3]  rep_seq_y=[0 0.0 0.6 0.8 0.8 0.6 0.3 0.1 0.0 0]
  Sum : Sum  Orientation=down  Inputs=++  SaturateOnIntegerOverflow=on
  out : Outport  Orientation=down  Port=1  InitialOutput=0
  wires:
  6 Saliences/1 -> Sum/1
  Constant/1 -> Mux/2
  Repeating Sequence/1 -> Mux/1
  Aux steps/1 -> Sum/2
  Sum/1 -> out/1

== system multi_opts/Saliences/step pairs ==
  Constant : Constant  Orientation=down  Value=[0 0 0 0]
  Mux : Mux  Orientation=down  Inputs=3
      settings: DisplayOption=none
  Repeating Sequence : simulink3/Sources/Repeating Sequence  Orientation=down  rep_seq_t=[0 0.5 1.0 1.5 2.0 2.5 3.0 3.5 4 4.5]  rep_seq_y=[0.2 0.3 0.4 0.5 0.6 0.7 0.8 0.9 1 1.1]
  Repeating Sequence1 : simulink3/Sources/Repeating Sequence  Orientation=down  rep_seq_t=[0 4.5 9 13.5 18 22.5 27 31.5 36 40.5]  rep_seq_y=[0.2 0.3 0.4 0.5 0.6 0.7 0.8 0.9 1 1.1]
  Scope : Scope
      settings: TickLabels=on  TimeRange=auto  YMin=-5  YMax=5  SaveToWorkspace=off  SaveName=ScopeData  DataFormat=Array  LimitDataPoints=on  MaxDataPoints=5000
  Zero-Order Hold : ZeroOrderHold  Orientation=down  SampleTime=0.5
  Zero-Order Hold1 : ZeroOrderHold  Orientation=down  SampleTime=4.5
  out : Outport  Orientation=down  Port=1  InitialOutput=0
  wires:
  Repeating Sequence/1 -> Zero-Order Hold/1
  Zero-Order Hold/1 -> Mux/1
  Zero-Order Hold1/1 -> Mux/2
  Repeating Sequence1/1 -> Zero-Order Hold1/1
  Mux/1 -> out/1, Scope/1
  Constant/1 -> Mux/3

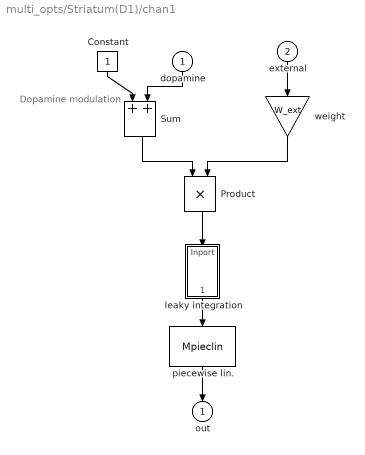
== system multi_opts/Striatum(D1)/chan1 ==
  note: Dopamine
      | modulation
  dopamine : Inport  Orientation=down  Port=1  LatchInput=off  PortDimensions=1
  external : Inport  Orientation=down  Port=2  LatchInput=off
  Constant : Constant  Orientation=down  Value=1
  Product : Product  Orientation=down  Inputs=2  Multiplication=Element-wise(.*)  SaturateOnIntegerOverflow=on
  Sum : Sum  Orientation=down  Inputs=++  SaturateOnIntegerOverflow=on
  leaky integration : Subsystem  Orientation=down
      settings: RTWFcnNameOpts=Auto  RTWFileNameOpts=Auto
  piecewise lin. : S-Function  Orientation=down  FunctionName=Mpieclin  Parameters=slope,thresh  PortCounts=[]  SFunctionModules=''
  weight : Gain  Orientation=down  Gain=W_ext  Multiplication=Element-wise(K.*u)  SaturateOnIntegerOverflow=on
  out : Outport  Orientation=down  Port=1  InitialOutput=0
  wires:
  weight/1 -> Product/2
  Product/1 -> leaky integration/1(Inport)
  Constant/1 -> Sum/1
  external/1 -> weight/1
  piecewise lin./1 -> out/1
  leaky integration/1(Outport) -> piecewise lin./1
  dopamine/1 -> Sum/2
  Sum/1 -> Product/1

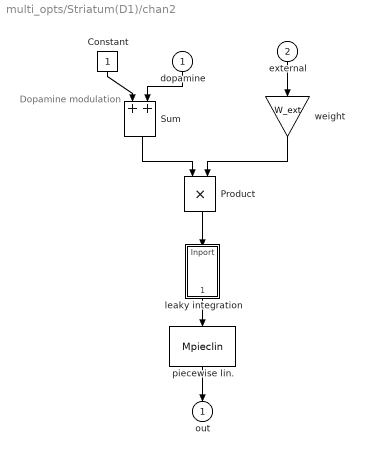
== system multi_opts/Striatum(D1)/chan2 ==
  note: Dopamine
      | modulation
  dopamine : Inport  Orientation=down  Port=1  LatchInput=off
  external : Inport  Orientation=down  Port=2  LatchInput=off
  Constant : Constant  Orientation=down  Value=1
  Product : Product  Orientation=down  Inputs=2  Multiplication=Element-wise(.*)  SaturateOnIntegerOverflow=on
  Sum : Sum  Orientation=down  Inputs=++  SaturateOnIntegerOverflow=on
  leaky integration : Subsystem  Orientation=down
      settings: RTWFcnNameOpts=Auto  RTWFileNameOpts=Auto
  piecewise lin. : S-Function  Orientation=down  FunctionName=Mpieclin  Parameters=slope,thresh  PortCounts=[]  SFunctionModules=''
  weight : Gain  Orientation=down  Gain=W_ext  Multiplication=Element-wise(K.*u)  SaturateOnIntegerOverflow=on
  out : Outport  Orientation=down  Port=1  InitialOutput=0
  wires:
  Sum/1 -> Product/1
  dopamine/1 -> Sum/2
  leaky integration/1(Outport) -> piecewise lin./1
  piecewise lin./1 -> out/1
  external/1 -> weight/1
  Constant/1 -> Sum/1
  Product/1 -> leaky integration/1(Inport)
  weight/1 -> Product/2

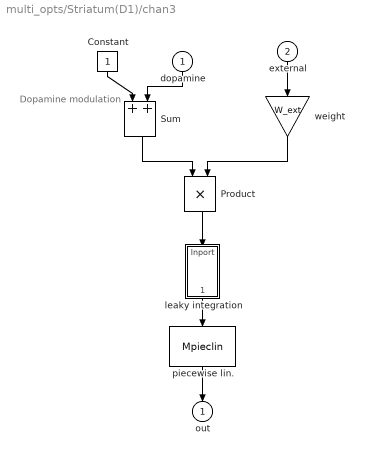
== system multi_opts/Striatum(D1)/chan3 ==
  note: Dopamine
      | modulation
  dopamine : Inport  Orientation=down  Port=1  LatchInput=off
  external : Inport  Orientation=down  Port=2  LatchInput=off
  Constant : Constant  Orientation=down  Value=1
  Product : Product  Orientation=down  Inputs=2  Multiplication=Element-wise(.*)  SaturateOnIntegerOverflow=on
  Sum : Sum  Orientation=down  Inputs=++  SaturateOnIntegerOverflow=on
  leaky integration : Subsystem  Orientation=down
      settings: RTWFcnNameOpts=Auto  RTWFileNameOpts=Auto
  piecewise lin. : S-Function  Orientation=down  FunctionName=Mpieclin  Parameters=slope,thresh  PortCounts=[]  SFunctionModules=''
  weight : Gain  Orientation=down  Gain=W_ext  Multiplication=Element-wise(K.*u)  SaturateOnIntegerOverflow=on
  out : Outport  Orientation=down  Port=1  InitialOutput=0
  wires:
  weight/1 -> Product/2
  Product/1 -> leaky integration/1(Inport)
  Constant/1 -> Sum/1
  external/1 -> weight/1
  piecewise lin./1 -> out/1
  leaky integration/1(Outport) -> piecewise lin./1
  dopamine/1 -> Sum/2
  Sum/1 -> Product/1

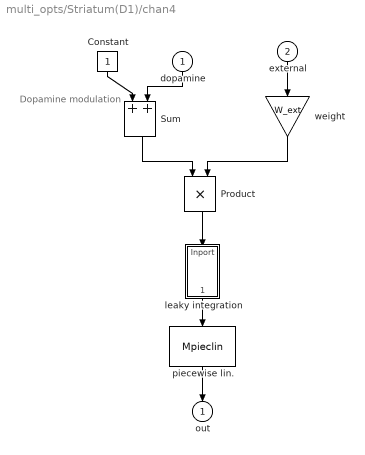
== system multi_opts/Striatum(D1)/chan4 ==
  note: Dopamine
      | modulation
  dopamine : Inport  Orientation=down  Port=1  LatchInput=off  PortDimensions=1
  external : Inport  Orientation=down  Port=2  LatchInput=off
  Constant : Constant  Orientation=down  Value=1
  Product : Product  Orientation=down  Inputs=2  Multiplication=Element-wise(.*)  SaturateOnIntegerOverflow=on
  Sum : Sum  Orientation=down  Inputs=++  SaturateOnIntegerOverflow=on
  leaky integration : Subsystem  Orientation=down
      settings: RTWFcnNameOpts=Auto  RTWFileNameOpts=Auto
  piecewise lin. : S-Function  Orientation=down  FunctionName=Mpieclin  Parameters=slope,thresh  PortCounts=[]  SFunctionModules=''
  weight : Gain  Orientation=down  Gain=W_ext  Multiplication=Element-wise(K.*u)  SaturateOnIntegerOverflow=on
  out : Outport  Orientation=down  Port=1  InitialOutput=0
  wires:
  Sum/1 -> Product/1
  dopamine/1 -> Sum/2
  leaky integration/1(Outport) -> piecewise lin./1
  piecewise lin./1 -> out/1
  external/1 -> weight/1
  Constant/1 -> Sum/1
  Product/1 -> leaky integration/1(Inport)
  weight/1 -> Product/2

== system multi_opts/Striatum(D1)/chan5 ==
  note: Dopamine
      | modulation
  dopamine : Inport  Orientation=down  Port=1  LatchInput=off
  external : Inport  Orientation=down  Port=2  LatchInput=off
  Constant : Constant  Orientation=down  Value=1
  Product : Product  Orientation=down  Inputs=2  Multiplication=Element-wise(.*)  SaturateOnIntegerOverflow=on
  Sum : Sum  Orientation=down  Inputs=++  SaturateOnIntegerOverflow=on
  leaky integration : Subsystem  Orientation=down
      settings: RTWFcnNameOpts=Auto  RTWFileNameOpts=Auto
  piecewise lin. : S-Function  Orientation=down  FunctionName=Mpieclin  Parameters=slope,thresh  PortCounts=[]  SFunctionModules=''
  weight : Gain  Orientation=down  Gain=W_ext  Multiplication=Element-wise(K.*u)  SaturateOnIntegerOverflow=on
  out : Outport  Orientation=down  Port=1  InitialOutput=0
  wires:
  weight/1 -> Product/2
  Product/1 -> leaky integration/1(Inport)
  Constant/1 -> Sum/1
  external/1 -> weight/1
  piecewise lin./1 -> out/1
  leaky integration/1(Outport) -> piecewise lin./1
  dopamine/1 -> Sum/2
  Sum/1 -> Product/1

== system multi_opts/Striatum(D1)/chan6 ==
  note: Dopamine
      | modulation
  dopamine : Inport  Orientation=down  Port=1  LatchInput=off
  external : Inport  Orientation=down  Port=2  LatchInput=off
  Constant : Constant  Orientation=down  Value=1
  Product : Product  Orientation=down  Inputs=2  Multiplication=Element-wise(.*)  SaturateOnIntegerOverflow=on
  Sum : Sum  Orientation=down  Inputs=++  SaturateOnIntegerOverflow=on
  leaky integration : Subsystem  Orientation=down
      settings: RTWFcnNameOpts=Auto  RTWFileNameOpts=Auto
  piecewise lin. : S-Function  Orientation=down  FunctionName=Mpieclin  Parameters=slope,thresh  PortCounts=[]  SFunctionModules=''
  weight : Gain  Orientation=down  Gain=W_ext  Multiplication=Element-wise(K.*u)  SaturateOnIntegerOverflow=on
  out : Outport  Orientation=down  Port=1  InitialOutput=0
  wires:
  Sum/1 -> Product/1
  dopamine/1 -> Sum/2
  leaky integration/1(Outport) -> piecewise lin./1
  piecewise lin./1 -> out/1
  external/1 -> weight/1
  Constant/1 -> Sum/1
  Product/1 -> leaky integration/1(Inport)
  weight/1 -> Product/2

== system multi_opts/Striatum(D2)/chan1 ==
  note: Dopamine
      | modulation
  dopamine : Inport  Orientation=down  Port=1  LatchInput=off  PortDimensions=1
  external : Inport  Orientation=down  Port=2  LatchInput=off
  Constant : Constant  Orientation=down  Value=1
  Product : Product  Orientation=down  Inputs=2  Multiplication=Element-wise(.*)  SaturateOnIntegerOverflow=on
  Sum : Sum  Orientation=down  Inputs=+-  SaturateOnIntegerOverflow=on
  leaky integration : Subsystem  Orientation=down
      settings: RTWFcnNameOpts=Auto  RTWFileNameOpts=Auto
  piecewise lin. : S-Function  Orientation=down  FunctionName=Mpieclin  Parameters=slope,thresh  PortCounts=[]  SFunctionModules=''
  weight : Gain  Orientation=down  Gain=W_ext  Multiplication=Element-wise(K.*u)  SaturateOnIntegerOverflow=on
  out : Outport  Orientation=down  Port=1  InitialOutput=0
  wires:
  Sum/1 -> Product/1
  dopamine/1 -> Sum/2
  leaky integration/1(Outport) -> piecewise lin./1
  piecewise lin./1 -> out/1
  external/1 -> weight/1
  Constant/1 -> Sum/1
  Product/1 -> leaky integration/1(Inport)
  weight/1 -> Product/2

== system multi_opts/Striatum(D2)/chan2 ==
  note: Dopamine
      | modulation
  dopamine : Inport  Orientation=down  Port=1  LatchInput=off  PortDimensions=1
  external : Inport  Orientation=down  Port=2  LatchInput=off
  Constant : Constant  Orientation=down  Value=1
  Product : Product  Orientation=down  Inputs=2  Multiplication=Element-wise(.*)  SaturateOnIntegerOverflow=on
  Sum : Sum  Orientation=down  Inputs=+-  SaturateOnIntegerOverflow=on
  leaky integration : Subsystem  Orientation=down
      settings: RTWFcnNameOpts=Auto  RTWFileNameOpts=Auto
  piecewise lin. : S-Function  Orientation=down  FunctionName=Mpieclin  Parameters=slope,thresh  PortCounts=[]  SFunctionModules=''
  weight : Gain  Orientation=down  Gain=W_ext  Multiplication=Element-wise(K.*u)  SaturateOnIntegerOverflow=on
  out : Outport  Orientation=down  Port=1  InitialOutput=0
  wires:
  weight/1 -> Product/2
  Product/1 -> leaky integration/1(Inport)
  Constant/1 -> Sum/1
  external/1 -> weight/1
  piecewise lin./1 -> out/1
  leaky integration/1(Outport) -> piecewise lin./1
  dopamine/1 -> Sum/2
  Sum/1 -> Product/1

== system multi_opts/Striatum(D2)/chan3 ==
  note: Dopamine
      | modulation
  dopamine : Inport  Orientation=down  Port=1  LatchInput=off  PortDimensions=1
  external : Inport  Orientation=down  Port=2  LatchInput=off
  Constant : Constant  Orientation=down  Value=1
  Product : Product  Orientation=down  Inputs=2  Multiplication=Element-wise(.*)  SaturateOnIntegerOverflow=on
  Sum : Sum  Orientation=down  Inputs=+-  SaturateOnIntegerOverflow=on
  leaky integration : Subsystem  Orientation=down
      settings: RTWFcnNameOpts=Auto  RTWFileNameOpts=Auto
  piecewise lin. : S-Function  Orientation=down  FunctionName=Mpieclin  Parameters=slope,thresh  PortCounts=[]  SFunctionModules=''
  weight : Gain  Orientation=down  Gain=W_ext  Multiplication=Element-wise(K.*u)  SaturateOnIntegerOverflow=on
  out : Outport  Orientation=down  Port=1  InitialOutput=0
  wires:
  Sum/1 -> Product/1
  dopamine/1 -> Sum/2
  leaky integration/1(Outport) -> piecewise lin./1
  piecewise lin./1 -> out/1
  external/1 -> weight/1
  Constant/1 -> Sum/1
  Product/1 -> leaky integration/1(Inport)
  weight/1 -> Product/2

== system multi_opts/Striatum(D2)/chan4 ==
  note: Dopamine
      | modulation
  dopamine : Inport  Orientation=down  Port=1  LatchInput=off  PortDimensions=1
  external : Inport  Orientation=down  Port=2  LatchInput=off
  Constant : Constant  Orientation=down  Value=1
  Product : Product  Orientation=down  Inputs=2  Multiplication=Element-wise(.*)  SaturateOnIntegerOverflow=on
  Sum : Sum  Orientation=down  Inputs=+-  SaturateOnIntegerOverflow=on
  leaky integration : Subsystem  Orientation=down
      settings: RTWFcnNameOpts=Auto  RTWFileNameOpts=Auto
  piecewise lin. : S-Function  Orientation=down  FunctionName=Mpieclin  Parameters=slope,thresh  PortCounts=[]  SFunctionModules=''
  weight : Gain  Orientation=down  Gain=W_ext  Multiplication=Element-wise(K.*u)  SaturateOnIntegerOverflow=on
  out : Outport  Orientation=down  Port=1  InitialOutput=0
  wires:
  weight/1 -> Product/2
  Product/1 -> leaky integration/1(Inport)
  Constant/1 -> Sum/1
  external/1 -> weight/1
  piecewise lin./1 -> out/1
  leaky integration/1(Outport) -> piecewise lin./1
  dopamine/1 -> Sum/2
  Sum/1 -> Product/1

== system multi_opts/Striatum(D2)/chan5 ==
  note: Dopamine
      | modulation
  dopamine : Inport  Orientation=down  Port=1  LatchInput=off  PortDimensions=1
  external : Inport  Orientation=down  Port=2  LatchInput=off
  Constant : Constant  Orientation=down  Value=1
  Product : Product  Orientation=down  Inputs=2  Multiplication=Element-wise(.*)  SaturateOnIntegerOverflow=on
  Sum : Sum  Orientation=down  Inputs=+-  SaturateOnIntegerOverflow=on
  leaky integration : Subsystem  Orientation=down
      settings: RTWFcnNameOpts=Auto  RTWFileNameOpts=Auto
  piecewise lin. : S-Function  Orientation=down  FunctionName=Mpieclin  Parameters=slope,thresh  PortCounts=[]  SFunctionModules=''
  weight : Gain  Orientation=down  Gain=W_ext  Multiplication=Element-wise(K.*u)  SaturateOnIntegerOverflow=on
  out : Outport  Orientation=down  Port=1  InitialOutput=0
  wires:
  Sum/1 -> Product/1
  dopamine/1 -> Sum/2
  leaky integration/1(Outport) -> piecewise lin./1
  piecewise lin./1 -> out/1
  external/1 -> weight/1
  Constant/1 -> Sum/1
  Product/1 -> leaky integration/1(Inport)
  weight/1 -> Product/2

== system multi_opts/Striatum(D2)/chan6 ==
  note: Dopamine
      | modulation
  dopamine : Inport  Orientation=down  Port=1  LatchInput=off  PortDimensions=1
  external : Inport  Orientation=down  Port=2  LatchInput=off
  Constant : Constant  Orientation=down  Value=1
  Product : Product  Orientation=down  Inputs=2  Multiplication=Element-wise(.*)  SaturateOnIntegerOverflow=on
  Sum : Sum  Orientation=down  Inputs=+-  SaturateOnIntegerOverflow=on
  leaky integration : Subsystem  Orientation=down
      settings: RTWFcnNameOpts=Auto  RTWFileNameOpts=Auto
  piecewise lin. : S-Function  Orientation=down  FunctionName=Mpieclin  Parameters=slope,thresh  PortCounts=[]  SFunctionModules=''
  weight : Gain  Orientation=down  Gain=W_ext  Multiplication=Element-wise(K.*u)  SaturateOnIntegerOverflow=on
  out : Outport  Orientation=down  Port=1  InitialOutput=0
  wires:
  weight/1 -> Product/2
  Product/1 -> leaky integration/1(Inport)
  Constant/1 -> Sum/1
  external/1 -> weight/1
  piecewise lin./1 -> out/1
  leaky integration/1(Outport) -> piecewise lin./1
  dopamine/1 -> Sum/2
  Sum/1 -> Product/1

== system multi_opts/GPe/2 input channel/input summation ==
  x1 : Inport  Port=1  LatchInput=off
  x2 : Inport  Port=2  LatchInput=off
  Sum : Sum  Inputs=++  SaturateOnIntegerOverflow=on
  W1 : Gain  Gain=W_str  Multiplication=Element-wise(K.*u)  SaturateOnIntegerOverflow=on
  W2 : Gain  Gain=W_STN  Multiplication=Element-wise(K.*u)  SaturateOnIntegerOverflow=on
  out_1 : Outport  Port=1  InitialOutput=0
  wires:
  W2/1 -> Sum/2
  W1/1 -> Sum/1
  x2/1 -> W2/1
  x1/1 -> W1/1
  Sum/1 -> out_1/1

== system multi_opts/GPe/2 input channel/leaky integration ==
  Inport : Inport  Port=1  LatchInput=off
  Gain : Gain  Gain=A_rate  Multiplication=Element-wise(K.*u)  SaturateOnIntegerOverflow=on
  Integrator : Integrator  ExternalReset=none  InitialConditionSource=internal  InitialCondition=0  LimitOutput=off  UpperSaturationLimit=inf  LowerSaturationLimit=-inf  ShowSaturationPort=off  ShowStatePort=off  AbsoluteTolerance=auto
  decay const : Gain  Orientation=left  Gain=-A_rate  Multiplication=Element-wise(K.*u)  SaturateOnIntegerOverflow=on
  sum : Sum  Inputs=++  SaturateOnIntegerOverflow=on
  Outport : Outport  Port=1  InitialOutput=0
  wires:
  Gain/1 -> sum/1
  Inport/1 -> Gain/1
  Integrator/1 -> decay const/1, Outport/1
  sum/1 -> Integrator/1
  decay const/1 -> sum/2

== system multi_opts/GPe/2 input channel1/input summation ==
  x1 : Inport  Port=1  LatchInput=off
  x2 : Inport  Port=2  LatchInput=off
  Sum : Sum  Inputs=++  SaturateOnIntegerOverflow=on
  W1 : Gain  Gain=W_str  Multiplication=Element-wise(K.*u)  SaturateOnIntegerOverflow=on
  W2 : Gain  Gain=W_STN  Multiplication=Element-wise(K.*u)  SaturateOnIntegerOverflow=on
  out_1 : Outport  Port=1  InitialOutput=0
  wires:
  Sum/1 -> out_1/1
  x1/1 -> W1/1
  x2/1 -> W2/1
  W1/1 -> Sum/1
  W2/1 -> Sum/2

== system multi_opts/GPe/2 input channel1/leaky integration ==
  Inport : Inport  Port=1  LatchInput=off
  Gain : Gain  Gain=A_rate  Multiplication=Element-wise(K.*u)  SaturateOnIntegerOverflow=on
  Integrator : Integrator  ExternalReset=none  InitialConditionSource=internal  InitialCondition=0  LimitOutput=off  UpperSaturationLimit=inf  LowerSaturationLimit=-inf  ShowSaturationPort=off  ShowStatePort=off  AbsoluteTolerance=auto
  decay const : Gain  Orientation=left  Gain=-A_rate  Multiplication=Element-wise(K.*u)  SaturateOnIntegerOverflow=on
  sum : Sum  Inputs=++  SaturateOnIntegerOverflow=on
  Outport : Outport  Port=1  InitialOutput=0
  wires:
  decay const/1 -> sum/2
  sum/1 -> Integrator/1
  Integrator/1 -> Outport/1, decay const/1
  Inport/1 -> Gain/1
  Gain/1 -> sum/1

== system multi_opts/GPe/2 input channel2/input summation ==
  x1 : Inport  Port=1  LatchInput=off
  x2 : Inport  Port=2  LatchInput=off
  Sum : Sum  Inputs=++  SaturateOnIntegerOverflow=on
  W1 : Gain  Gain=W_str  Multiplication=Element-wise(K.*u)  SaturateOnIntegerOverflow=on
  W2 : Gain  Gain=W_STN  Multiplication=Element-wise(K.*u)  SaturateOnIntegerOverflow=on
  out_1 : Outport  Port=1  InitialOutput=0
  wires:
  W2/1 -> Sum/2
  W1/1 -> Sum/1
  x2/1 -> W2/1
  x1/1 -> W1/1
  Sum/1 -> out_1/1

== system multi_opts/GPe/2 input channel2/leaky integration ==
  Inport : Inport  Port=1  LatchInput=off
  Gain : Gain  Gain=A_rate  Multiplication=Element-wise(K.*u)  SaturateOnIntegerOverflow=on
  Integrator : Integrator  ExternalReset=none  InitialConditionSource=internal  InitialCondition=0  LimitOutput=off  UpperSaturationLimit=inf  LowerSaturationLimit=-inf  ShowSaturationPort=off  ShowStatePort=off  AbsoluteTolerance=auto
  decay const : Gain  Orientation=left  Gain=-A_rate  Multiplication=Element-wise(K.*u)  SaturateOnIntegerOverflow=on
  sum : Sum  Inputs=++  SaturateOnIntegerOverflow=on
  Outport : Outport  Port=1  InitialOutput=0
  wires:
  Gain/1 -> sum/1
  Inport/1 -> Gain/1
  Integrator/1 -> decay const/1, Outport/1
  sum/1 -> Integrator/1
  decay const/1 -> sum/2

== system multi_opts/GPe/2 input channel3/input summation ==
  x1 : Inport  Port=1  LatchInput=off
  x2 : Inport  Port=2  LatchInput=off
  Sum : Sum  Inputs=++  SaturateOnIntegerOverflow=on
  W1 : Gain  Gain=W_str  Multiplication=Element-wise(K.*u)  SaturateOnIntegerOverflow=on
  W2 : Gain  Gain=W_STN  Multiplication=Element-wise(K.*u)  SaturateOnIntegerOverflow=on
  out_1 : Outport  Port=1  InitialOutput=0
  wires:
  Sum/1 -> out_1/1
  x1/1 -> W1/1
  x2/1 -> W2/1
  W1/1 -> Sum/1
  W2/1 -> Sum/2
